simulink model "Simulation_in_Simulink"  (R2021b)
settings: Solver=FixedStepAuto  StartTime=0.0  StopTime=10  FixedStep=0.02  RelTol=1e-3
(part 4 of 5)

== matlab function Simulation_in_Simulink/MATLAB Function ==
  data: M input; C_theta_dot input; G input; taw input; theta_ddot output
function theta_ddot = fcn( M, C_theta_dot, G, taw)

MM=M;
CC=C_theta_dot;
GG=G;
torque=taw;


theta_ddot=MM\(torque- CC - GG);

end

== matlab function Simulation_in_Simulink/G ==
  data: theta input; G output
function G = fcn(theta)
 
g=9.81; % [m/s^2]

t2=theta(2);
t3=theta(3);
t4=theta(4);
t5=theta(5);
t6=theta(6);

a2=0.6129;
a3=0.5716;  
d5=0.1157; 
d6=0.0922;

G =[
 
                                                                                                                                                                                                                                                                                                                              0;
(g*(163280000*cos(t2 + t3) - 210469*sin(t2 + t3 + t4) + 294000000*cos(t2) + 582539*cos(t2 + t3 + t4)*sin(t5) + 20425*sin(t2 + t3 + t4)*cos(t6) + 218200000*a3*cos(t2 + t3) + 846200000*a2*cos(t2) - 119850000*d5*sin(t2 + t3 + t4) + 20425*cos(t2 + t3 + t4)*cos(t5)*sin(t6) + 21500000*d6*cos(t2 + t3 + t4)*sin(t5)))/50000000;
                                           (g*(163280000*cos(t2 + t3) - 210469*sin(t2 + t3 + t4) + 582539*cos(t2 + t3 + t4)*sin(t5) + 20425*sin(t2 + t3 + t4)*cos(t6) + 218200000*a3*cos(t2 + t3) - 119850000*d5*sin(t2 + t3 + t4) + 20425*cos(t2 + t3 + t4)*cos(t5)*sin(t6) + 21500000*d6*cos(t2 + t3 + t4)*sin(t5)))/50000000;
                                                                                                (g*(582539*cos(t2 + t3 + t4)*sin(t5) - 210469*sin(t2 + t3 + t4) + 20425*sin(t2 + t3 + t4)*cos(t6) - 119850000*d5*sin(t2 + t3 + t4) + 20425*cos(t2 + t3 + t4)*cos(t5)*sin(t6) + 21500000*d6*cos(t2 + t3 + t4)*sin(t5)))/50000000;
                                                                                                                                                                                                                                  (g*sin(t2 + t3 + t4)*(582539*cos(t5) - 20425*sin(t5)*sin(t6) + 21500000*d6*cos(t5)))/50000000;
                                                                                                                                                                                                                               (43*g*((19*cos(t2 + t3 + t4)*sin(t6))/20000 + (19*sin(t2 + t3 + t4)*cos(t5)*cos(t6))/20000))/100];
 


end
